simulink model "HCM"  (R2020a)
settings: Solver=VariableStepAuto  StartTime=0.0  StopTime=10.0  RelTol=1e-3
values from neighbouring files (symbols this model uses):
  a = 0.9    [halfcar.m]
  b = 1.2    [halfcar.m]
  Cf = 2500    [halfcar.m]
  Cr = 2000    [halfcar.m]
  I = 2100    [halfcar.m]
  kf = 28000    [halfcar.m]
  kr = 21000    [halfcar.m]
  ms = 12    [Constants.m]    (also in halfcar.m = 1356.65)
  muf = 67.835    [halfcar.m]
  mur = 67.835    [halfcar.m]
settings Model: Creator=sammy  LastModifiedBy=monal
settings DebuggingCC: SFMachineParentedDataDiag=error

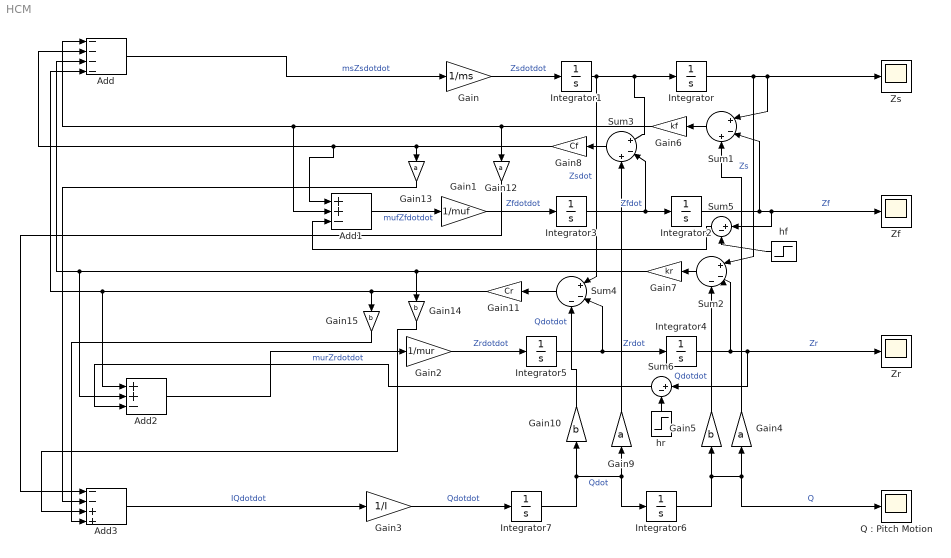
== system HCM ==
  Add : Sum  Inputs=----
  Add1 : Sum  Inputs=++-
  Add2 : Sum  Inputs=++-
  Add3 : Sum  Inputs=--++
  Gain : Gain  Gain=1/ms
  Gain1 : Gain  Gain=1/muf
  Gain{5,10,14..15} (4 alike) : Gain  Gain=b
  Gain11 : Gain  Gain=Cr
  Gain{4,9,12..13} (4 alike) : Gain  Gain=a
  Gain2 : Gain  Gain=1/mur
  Gain3 : Gain  Gain=1/I
  Gain6 : Gain  Gain=kf
  Gain7 : Gain  Gain=kr
  Gain8 : Gain  Gain=Cf
  Integrator{,1..7} (8 alike) : Integrator
  "Q : Pitch Motion" : Scope
  Sum1 : Sum  Inputs=|+-+
  Sum2 : Sum  Inputs=|+--
  Sum3 : Sum  Inputs=|+-+
  Sum4 : Sum  Inputs=|+--
  Sum5 : Sum  Inputs=|+-
  Sum6 : Sum  Inputs=|+-
  Zf : Scope
  Zr : Scope
  Zs : Scope
  hf : Step  After=0.03  SampleTime=0
  hr : Step  After=0.03  SampleTime=0
  wires:
  Integrator/1 -> Sum2/1, Sum1/1, Zs/1  "Zs"
  Integrator1/1 -> Sum3/1, Integrator/1, Sum4/1  "Zsdot"
  Gain/1 -> Integrator1/1  "Zsdotdot"
  Add/1 -> Gain/1  "msZsdotdot"
  Add1/1 -> Gain1/1  "mufZfdotdot"
  Integrator3/1 -> Sum3/2, Integrator2/1  "Zfdot"
  Integrator2/1 -> Sum1/2, Sum5/1, Zf/1  "Zf"
  Gain1/1 -> Integrator3/1  "Zfdotdot"
  Add2/1 -> Gain2/1  "murZrdotdot"
  Integrator5/1 -> Sum4/2, Integrator4/1  "Zrdot"
  Integrator4/1 -> Sum2/2, Sum6/1, Zr/1  "Zr"
  Gain2/1 -> Integrator5/1  "Zrdotdot"
  Add3/1 -> Gain3/1  "IQdotdot"
  Integrator6/1 -> Gain5/1, Gain4/1, "Q : Pitch Motion"/1  "Q"
  Gain3/1 -> Integrator7/1  "Qdotdot"
  Gain4/1 -> Sum1/3
  Sum1/1 -> Gain6/1
  Gain6/1 -> Gain12/1, Add1/2, Add/1
  Gain5/1 -> Sum2/3  "Qdotdot"
  Gain7/1 -> Add2/2, Add/3, Gain14/1
  Sum3/1 -> Gain8/1
  Integrator7/1 -> Integrator6/1, Gain9/1, Gain10/1  "Qdot"
  Gain9/1 -> Sum3/3
  Gain8/1 -> Gain13/1, Add1/1, Add/2
  Sum2/1 -> Gain7/1
  Gain10/1 -> Sum4/3  "Qdotdot"
  Sum4/1 -> Gain11/1
  Gain11/1 -> Gain15/1, Add2/1, Add/4
  hf/1 -> Sum5/2
  Sum5/1 -> Add1/3
  hr/1 -> Sum6/2
  Sum6/1 -> Add2/3
  Gain12/1 -> Add3/1
  Gain13/1 -> Add3/2
  Gain14/1 -> Add3/3
  Gain15/1 -> Add3/4
